simulink model "SimplePendulumMotion"  (R2021a)
settings: Solver=VariableStepAuto  StartTime=0.0  StopTime=10.0  MaxStep=1e-3  RelTol=1e-3
values from neighbouring files (symbols this model uses):
  g = 9.81    [SimplePendulumMotion_int.m]
  L = lengthValues(i)    [SimplePendulumMotion_int.m]
settings Model: Creator=lenovo  LastModifiedBy=lenovo

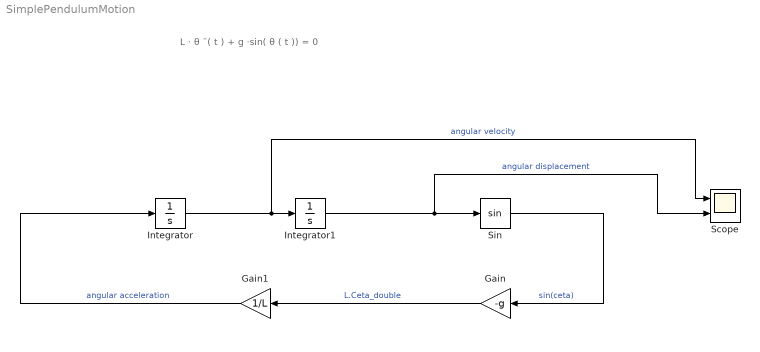
== system SimplePendulumMotion ==
  note: L ⋅ θ ¨( t ) + g ⋅sin( θ ( t )) = 0
  Gain : Gain  Gain=-g
  Gain1 : Gain  Gain=1/L
  Integrator : Integrator
  Integrator1 : Integrator  InitialCondition=2
  Scope : Scope  NumInputPorts=2
  Sin : Trigonometry
  wires:
  Gain1/1 -> Integrator/1  "angular acceleration"
  Integrator/1 -> Scope/1, Integrator1/1  "angular velocity"
  Integrator1/1 -> Scope/2, Sin/1  "angular displacement"
  Sin/1 -> Gain/1  "sin(ceta)"
  Gain/1 -> Gain1/1  "L.Ceta_double"
